simulink model "sim_slfbrd"  (R2013a)
settings: Solver=ode45  StartTime=0.0  StopTime=50  RelTol=1e-3
settings Model: Creator=Aleksandr  LastModifiedBy=Aleksandr

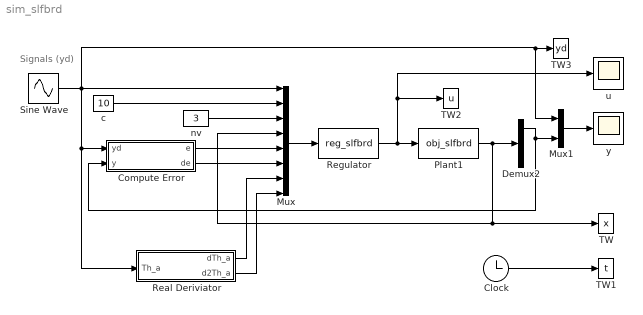
== system sim_slfbrd ==
  note: Signals (yd)
  Clock : Clock
      settings: Decimation=30
  "Compute Error " : Subsystem
  Demux2 : Demux  Outputs=3
  Mux : Mux  Inputs=8
  Mux1 : Mux  Inputs=2
  Plant1 : S-Function  FunctionName=obj_slfbrd  EnableBusSupport=off
  Real Deriviator : Subsystem
  Regulator : S-Function  FunctionName=reg_slfbrd  EnableBusSupport=off
  Sine Wave : Sin  SampleTime=0
  TW : ToWorkspace  VariableName=x  SampleTime=-1
  TW1 : ToWorkspace  VariableName=t  SampleTime=-1
  TW2 : ToWorkspace  VariableName=u  SampleTime=-1
  TW3 : ToWorkspace  VariableName=yd  SampleTime=-1
  c : Constant  Value=10
  nv : Constant  Value=3
  u : Scope
  y : Scope
  wires:
  c/1 -> Mux/2
  nv/1 -> Mux/3
  Mux/1 -> Regulator/1
  Regulator/1 -> TW2/1, u/1, Plant1/1
  Plant1/1 -> Demux2/1, Mux/4, TW/1
  Sine Wave/1 -> Real Deriviator/1(Th_a), "Compute Error "/1(yd), Mux1/1, TW3/1, Mux/1
  Real Deriviator/1(dTh_a) -> Mux/7
  Real Deriviator/2(d2Th_a) -> Mux/8
  Clock/1 -> TW1/1
  "Compute Error "/1(e) -> Mux/5
  "Compute Error "/2(de) -> Mux/6
  Demux2/1 -> Mux1/2, "Compute Error "/2(y)
  Mux1/1 -> y/1

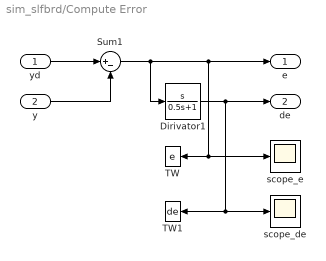
== system sim_slfbrd/Compute Error  ==
  yd : Inport
  y : Inport  Port=2
  Dirivator1 : TransferFcn  Numerator=[1 0]  Denominator=[0.5 1]
  Sum1 : Sum  Inputs=|+-
  TW : ToWorkspace  VariableName=e  SampleTime=-1
  TW1 : ToWorkspace  VariableName=de  SampleTime=-1
  scope_de : Scope
      settings: SaveName=ScopeData3
  scope_e : Scope
      settings: SaveName=ScopeData2
  e : Outport
  de : Outport  Port=2
  wires:
  yd/1 -> Sum1/1
  Sum1/1 -> Dirivator1/1, TW/1, scope_e/1, e/1
  y/1 -> Sum1/2
  Dirivator1/1 -> scope_de/1, TW1/1, de/1

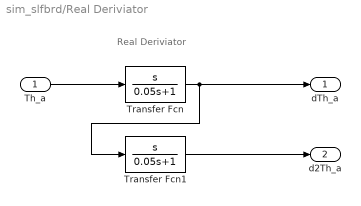
== system sim_slfbrd/Real Deriviator ==
  note: Real Deriviator
  Th_a : Inport
  Transfer Fcn : TransferFcn  Numerator=[1 0]  Denominator=[0.05 1]
  Transfer Fcn1 : TransferFcn  Numerator=[1 0]  Denominator=[0.05 1]
  dTh_a : Outport
  d2Th_a : Outport  Port=2
  wires:
  Transfer Fcn/1 -> dTh_a/1, Transfer Fcn1/1
  Th_a/1 -> Transfer Fcn/1
  Transfer Fcn1/1 -> d2Th_a/1
